simulink model "expt_5_d"  (R2018b)
settings: Solver=VariableStepAuto  StartTime=0.0  StopTime=0.1  RelTol=1e-3
libraries: commfilt2 x1, commrandsrc3 x1
settings Model: Creator=sangh  LastModifiedBy=sangh

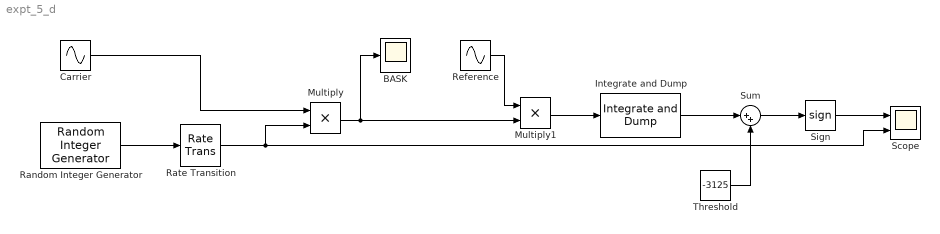
== system expt_5_d ==
  BASK : Scope
  Carrier : Sin  Amplitude=5  Frequency=20e3  SampleTime=2e-6
  Integrate and Dump : commfilt2/Integrate and Dump  obssamples=500  offsetsamples=0  nodump=off  roundingMode=Floor  overflowMode=off  outputDataTypeStr=Inherit: Same as accumulator  outputLastDataTypeStr=Inherit: Same as accumulator
      settings: SourceProductName=Communications System Toolbox
  Multiply : Product
  Multiply1 : Product
  Random Integer Generator : commrandsrc3/Random Integer Generator  SetSize=2  SeedSource=Auto  Seed=0  SampleTime=0.001  SamplesPerFrame=1  OutputDataType=boolean  SimulateUsing=Interpreted execution
  Rate Transition : RateTransition  OutPortSampleTime=2e-6
  Reference : Sin  Amplitude=5  Frequency=20e3  SampleTime=2e-6
  Scope : Scope  NumInputPorts=2
  Sign : Signum
  Sum : Sum  Inputs=|++
  "Threshold " : Constant  Value=-3125
  wires:
  Carrier/1 -> Multiply/1
  Rate Transition/1 -> Scope/2, Multiply/2
  Multiply/1 -> Multiply1/2, BASK/1
  Random Integer Generator/1 -> Rate Transition/1
  Reference/1 -> Multiply1/1
  Multiply1/1 -> Integrate and Dump/1
  Integrate and Dump/1 -> Sum/1
  "Threshold "/1 -> Sum/2
  Sum/1 -> Sign/1
  Sign/1 -> Scope/1
